simulink model "NonlinearValveWithGainChange"  (R2013b)
settings: Solver=ode45  StartTime=0.0  StopTime=400  RelTol=1e-3
settings Model: Creator=MMSA  LastModifiedBy=MMSA
settings SolverCC: ZeroCrossAlgorithm=Adaptive  PositivePriorityOrder=on
settings HardwareCC: ProdBitPerPointer=64  ProdHWDeviceType=Generic->64-bit Embedded Processor (LLP64)

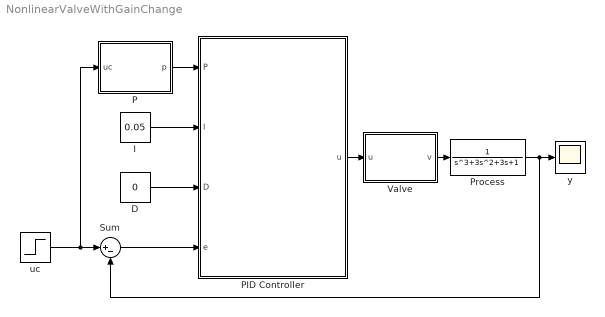
== system NonlinearValveWithGainChange ==
  D : Constant  Value=0
  I : Constant  Value=0.05
  P : MATLAB Function  TreatAsAtomicUnit=on
  PID Controller : Subsystem
  Process : TransferFcn  Denominator=[1 3 3 1]  AbsoluteTolerance=-1
  Sum : Sum  Inputs=|+-
  Valve : MATLAB Function  TreatAsAtomicUnit=on
  uc : Step  Time=200  Before=5  After=5.1  SampleTime=0
  y : Scope
      settings: TimeRange=7000  YMin=0
  wires:
  Valve/1(v) -> Process/1
  PID Controller/1(u) -> Valve/1(u)
  Sum/1 -> PID Controller/4(e)
  Process/1 -> Sum/2, y/1
  uc/1 -> Sum/1, P/1(uc)
  D/1 -> PID Controller/3(D)
  I/1 -> PID Controller/2(I)
  P/1(p) -> PID Controller/1(P)

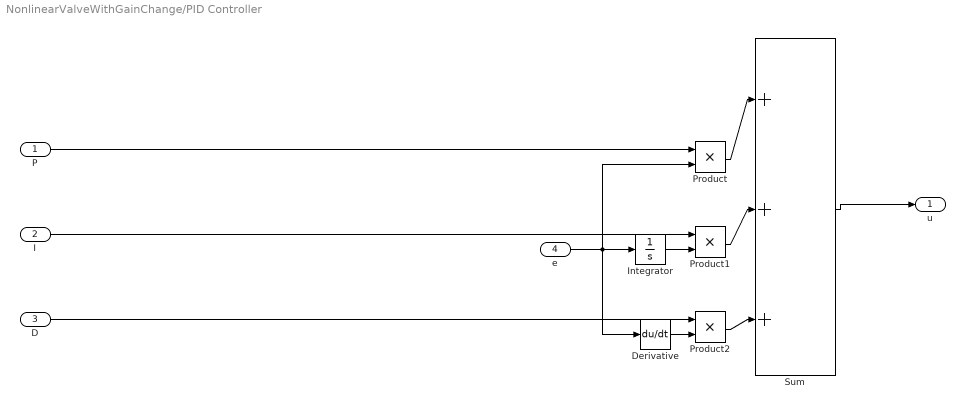
== system NonlinearValveWithGainChange/PID Controller ==
  P : Inport
  I : Inport  Port=2
  D : Inport  Port=3
  e : Inport  Port=4
  Derivative : Derivative
  Integrator : Integrator
  Product : Product
  Product1 : Product
  Product2 : Product
  Sum : Sum  Inputs=|+++
  u : Outport
  wires:
  I/1 -> Product1/1
  P/1 -> Product/1
  Sum/1 -> u/1
  D/1 -> Product2/1
  Product/1 -> Sum/1
  e/1 -> Derivative/1, Product/2, Integrator/1
  Integrator/1 -> Product1/2
  Product2/1 -> Sum/3
  Derivative/1 -> Product2/2
  Product1/1 -> Sum/2

== matlab function NonlinearValveWithGainChange/P ==
  data: uc input; p output
function p  = P(uc)
if uc < 1
    p=uc;
else
    p=1/uc;
end

== matlab function NonlinearValveWithGainChange/Valve ==
  data: u input; v output
function v = Valve(u)
v=u^4;
end
